simulink model "RL_Traction_motor"  (R2023a)
settings: Solver=VariableStepAuto  StartTime=0.0  StopTime=0.25  RelTol=1e-3
model workspace (MAT data in the model file):
  Cdc = 0.001
  Jm = 0.1234
  Ki_id = 710.3004
  Ki_iq = 1061.5
  Ki_omega = 500
  Kp_id = 0.8779
  Kp_iq = 1.0744
  Kp_omega = 20
  L0 = 0.00012184
  Ld = 0.00024368
  LdMatrix = [0.000182 0.00018 0.000178 0.000177 0.000176 0.00017475 0.0001735 0.00017247 0.00017132 0.00016571 0.00016537 0.00016571 ... (735 elements, 21x35)]
  Lq = 0.00029758
  LqMatrix = [0.000217 0.000217 0.000217 0.000217 0.000217 0.0002145 0.000212 0.0002115 0.00021022 0.0002079 0.00020461 0.0002079 ... (735 elements, 21x35)]
  PmMatrix = [0.0363 0.0363 0.0363 0.0363 0.0363 0.0363 0.0363 0.0363 0.0363 0.0363 0.0363 0.0363 ... (735 elements, 21x35)]
  Pmax = 35000
  Rs = 0.010087
  Tmax = 200
  Ts = 5e-06
  Tsc = 0.0001
  V1 = 290
  Vnom = 325
  fsw = 10000
  idVec = [-250 -225 -200 -175 -150 -125 -100 -75 -50 -25 0 25 ... (21 elements, 1x21)]
  iqVec = [-425 -400 -375 -350 -325 -300 -275 -250 -225 -200 -175 -150 ... (35 elements, 1x35)]
  p = 8
  psim = 0.044
undefined symbols (not defined in the file or in its folder): ee_sli_rtmsupport, gcbh, idMatrix, Imax, iqMatrix, rpmVec, TqVec, VdcVec
libraries: fl_lib x19, nesl_utility x13, eeGeneralControl x9, slpidlib x7, ee_lib x6, simulink x3, eeTransforms x2, batteryecm_lib x1, eeDqVoltageLimiter x1, eePwmGeneratorTwoLevel x1, eeResolverToDigitalConverter x1
(part 2 of 3)

== system RL_Traction_motor/Sensing Vdc ==
  PS-Simulink Converter4 : nesl_utility/PS-Simulink Converter  PhysicalDomain=network_engine_domain  SubClassName=ps_output  LeftPortType=input  RightPortType=output  PseudoPeriodic=off  Frequencies=[]  VectorFormat=1-D array  Unit=V  AffineConversion=off
  Voltage Sensor : fl_lib/Electrical/Electrical Sensors/Voltage Sensor
  + : PMIOPort  Side=Left
  - : PMIOPort  Port=2  Side=Right
  tag scope: Vdc=global
  wires:
  PS-Simulink Converter4/1 -> [Vdc]
  connections:
  Voltage Sensor/LConn1 -- +/RConn1
  Voltage Sensor/RConn2 -- -/RConn1
  PS-Simulink Converter4/LConn1 -- Voltage Sensor/RConn1

== system RL_Traction_motor/Sensing iabc ==
  Current Sensor : ee_lib/Sensors & Transducers/Current Sensor (Three-Phase)
      settings: LogSimulationData=on
  PS-Simulink Converter : nesl_utility/PS-Simulink Converter  PhysicalDomain=network_engine_domain  SubClassName=ps_output  LeftPortType=input  RightPortType=output  PseudoPeriodic=off  Frequencies=[]  VectorFormat=1-D array  Unit=A  AffineConversion=off
  Sensor time lag : Subsystem  mask{Ti=1e-5}
      mask prompts: Ti "Sensor time constant:"
  1 : PMIOPort  Side=Left
  2 : PMIOPort  Port=2  Side=Right
  tag scope: iabc=global
  wires:
  PS-Simulink Converter/1 -> Sensor time lag/1(In1)
  Sensor time lag/1(Out1) -> [iabc]
  connections:
  1/RConn1 -- Current Sensor/LConn1
  2/RConn1 -- Current Sensor/RConn2
  Current Sensor/RConn1 -- PS-Simulink Converter/LConn1

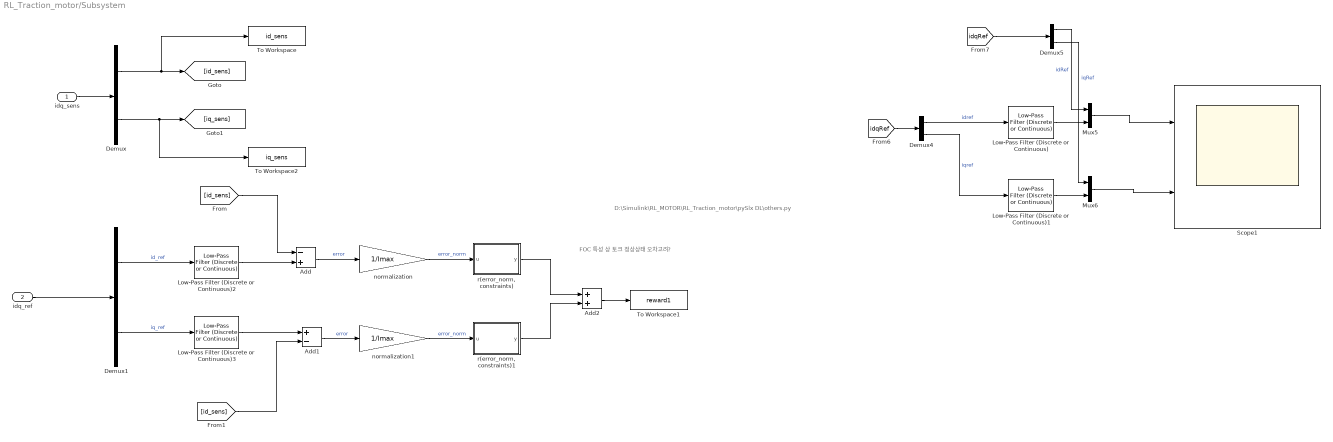
== system RL_Traction_motor/Subsystem ==
  note: D:\Simulink\RL_MOTOR\RL_Traction_motor\pySlx DL\others.py
  note: FOC 특성 상 토크 정상상태 오차고려?
  idq_sens : Inport
  idq_ref : Inport  Port=2
  Add : Sum  Inputs=-+
  Add1 : Sum  Inputs=+-
  Add2 : Sum
  Demux{,1,4..5} (4 alike) : Demux  Outputs=2
  Low-Pass Filter (Discrete or Continuous) : eeGeneralControl/Low-Pass Filter (Discrete or Continuous)  K=1  T=2.776235e-4  B=inf  A=-inf  init_option=Inherited from block input  x0=0  Ts=-1
  Low-Pass Filter (Discrete or Continuous)1 : eeGeneralControl/Low-Pass Filter (Discrete or Continuous)  K=1  T=1/2338913  B=inf  A=-inf  init_option=Inherited from block input  x0=0  Ts=-1
  Low-Pass Filter (Discrete or Continuous)2 : eeGeneralControl/Low-Pass Filter (Discrete or Continuous)  K=1  T=2.776235e-4  B=inf  A=-inf  init_option=Inherited from block input  x0=0  Ts=-1
  Low-Pass Filter (Discrete or Continuous)3 : eeGeneralControl/Low-Pass Filter (Discrete or Continuous)  K=1  T=1/2338913  B=inf  A=-inf  init_option=Inherited from block input  x0=0  Ts=-1
  Mux5 : Mux  Inputs=2
  Mux6 : Mux  Inputs=2
  Scope1 : Scope  NumInputPorts=2
  To Workspace : ToWorkspace  VariableName=id_sens  SaveFormat=Timeseries  SampleTime=-1
  To Workspace1 : ToWorkspace  VariableName=reward1  SaveFormat=Timeseries  SampleTime=-1
  To Workspace2 : ToWorkspace  VariableName=iq_sens  SaveFormat=Timeseries  SampleTime=-1
  normalization : Gain  Gain=1/Imax
  normalization1 : Gain  Gain=1/Imax
  "r(error_norm, constraints)" : MATLAB Function  TreatAsAtomicUnit=on
  "r(error_norm, constraints)1" : MATLAB Function  TreatAsAtomicUnit=on
  wires:
  Mux5/1 -> Scope1/1
  Demux5/1 -> Mux5/1  "idRef"
  Low-Pass Filter (Discrete or Continuous)1/1 -> Mux6/2
  Mux6/1 -> Scope1/2
  Demux4/1 -> Low-Pass Filter (Discrete or Continuous)/1  "idref"
  [idqRef] -> Demux4/1
  Low-Pass Filter (Discrete or Continuous)/1 -> Mux5/2
  [idqRef] -> Demux5/1
  Demux4/2 -> Low-Pass Filter (Discrete or Continuous)1/1  "iqref"
  Demux5/2 -> Mux6/1  "iqRef"
  idq_sens/1 -> Demux/1
  idq_ref/1 -> Demux1/1
  Demux1/1 -> Low-Pass Filter (Discrete or Continuous)2/1  "id_ref"
  Demux1/2 -> Low-Pass Filter (Discrete or Continuous)3/1  "iq_ref"
  Demux/1 -> To Workspace/1, [id_sens]
  Demux/2 -> To Workspace2/1, [iq_sens]
  Low-Pass Filter (Discrete or Continuous)2/1 -> Add/2
  Low-Pass Filter (Discrete or Continuous)3/1 -> Add1/1
  Add/1 -> normalization/1  "error"
  normalization/1 -> "r(error_norm, constraints)"/1(u)  "error_norm"
  "r(error_norm, constraints)1"/1(y) -> Add2/2
  normalization1/1 -> "r(error_norm, constraints)1"/1(u)  "error_norm"
  Add1/1 -> normalization1/1  "error"
  Add2/1 -> To Workspace1/1
  "r(error_norm, constraints)"/1(y) -> Add2/1
  [id_sens] -> Add/1
  [id_sens] -> Add1/2

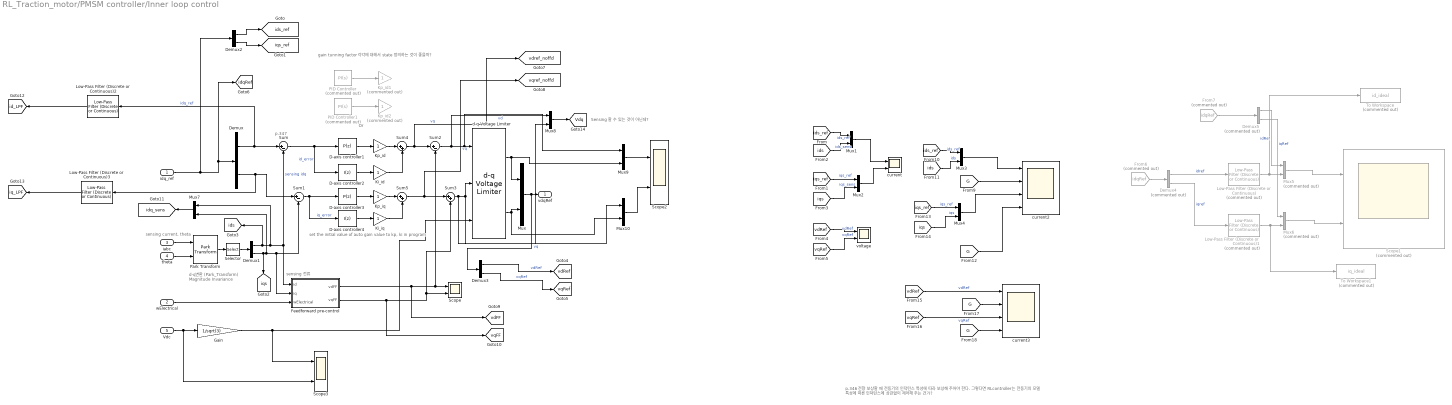
== system RL_Traction_motor/PMSM controller/Inner loop control ==
  note: Sensing 할 수 있는 것이 아닌데?
  note: gain tunning factor 각각에 대해서 state 정의하는 것이 좋을까?
  note: Or
  note: set the initial value of auto gain value to kp, ki in program
  note: p.346 전향 보상할 때 전동기의 인덕턴스 특성에 따라 보상해 주어야 한다.
      | 그렇다면 RLcontroller는 전동기의 모델 특성에 따른 인덕턴스에 상관없이 제어해 주는 건가?
  note: sensing current, theta
  note: p.347
  note: d-q변환
      | (Park_Transform)
      | Magnitude Invariance
  note: sensing 전류
  idq_ref : Inport
  wElectrical : Inport  Port=2
  iabc : Inport  Port=3
  theta : Inport  Port=4
  Vdc : Inport  Port=5
  D-axis controller1 : slpidlib/PID Controller  Controller=P  Form=Parallel  TimeDomain=Discrete-time  UseExternalTs=off  SampleTime=Tsc  IntegratorMethod=Forward Euler  FilterMethod=Forward Euler  ControllerParametersSource=internal  P=Kp_id  I="710.3          %710.3 (Ki_id)"  UseKiTs=off  D=0  N=100  UseFilter=on  TunerSelectOption=Transfer Function Based (PID Tuner App)  InitialConditionSource=internal  InitialConditionForIntegrator=0  InitialConditionForFilter=0  DifferentiatorICPrevScaledInput=0  ExternalReset=none  TrackingMode=off  Kt=1  LimitOutput=on  SatLimitsSource=internal  UpperSaturationLimit=Vnom/sqrt(3)  LowerSaturationLimit=-Vnom/sqrt(3)  LinearizeAsGain=on  AntiWindupMode=back-calculation  Kb=1000  LimitIntegrator=off  UpperIntegratorSaturationLimit=inf  LowerIntegratorSaturationLimit=-inf  POutMin=[]  POutMax=[]  IOutMin=[]  IOutMax=[]  DOutMin=[]  DOutMax=[]  NOutMin=[]  NOutMax=[]  SumOutMin=[]  SumOutMax=[]  SaturationOutMin=[]  SaturationOutMax=[]  PParamMin=[]  PParamMax=[]  IParamMin=[]  IParamMax=[]  DParamMin=[]  DParamMax=[]  NParamMin=[]  NParamMax=[]  KbParamMin=[]  KbParamMax=[]  KtParamMin=[]  KtParamMax=[]  KbOutMin=[]  KbOutMax=[]  KtOutMin=[]  KtOutMax=[]  IntegratorOutMin=[]  IntegratorOutMax=[]  FilterOutMin=[]  FilterOutMax=[]  SumI1OutMin=[]  SumI1OutMax=[]  SumI2OutMin=[]  SumI2OutMax=[]  SumI3OutMin=[]  SumI3OutMax=[]  SumI4OutMin=[]  SumI4OutMax=[]  SumDOutMin=[]  SumDOutMax=[]  DifferentiatorOutMin=[]  DifferentiatorOutMax=[]  FilterDiffOutCoefMin=[]  FilterDiffOutCoefMax=[]  ReciprocalOutMin=[]  ReciprocalOutMax=[]  SumDenOutMin=[]  SumDenOutMax=[]  SumNumOutMin=[]  SumNumOutMax=[]  DivideOutMin=[]  DivideOutMax=[]  UdiffTsProdOutMin=[]  UdiffTsProdOutMax=[]  NTsProdOutMin=[]  NTsProdOutMax=[]  UintegralTsProdOutMin=[]  UintegralTsProdOutMax=[]  UngainTsProdOutMin=[]  UngainTsProdOutMax=[]  ClampingZeroOutDataTypeStr=Inherit: Inherit via back propagation  ClampingZeroOutMin=[]  ClampingZeroOutMax=[]  FilterDenConstantOutDataTypeStr=Inherit: Inherit via back propagation  FilterDenConstantOutMin=[]  FilterDenConstantOutMax=[]  PCopyOutDataTypeStr=Inherit: Inherit via back propagation  PCopyOutMin=[]  PCopyOutMax=[]  NCopyOutDataTypeStr=Inherit: Inherit via back propagation  NCopyOutMin=[]  NCopyOutMax=[]  IntegratorContinuousStateAttributes=''  IntegratorStateMustResolveToSignalObject=off  IntegratorRTWStateStorageClass=Auto  FilterContinuousStateAttributes=''  FilterStateMustResolveToSignalObject=off  FilterRTWStateStorageClass=Auto  ParallelPVariant=InternalParameters  IdealPVariant=Disabled  IVariant=Disabled  DVariant=Disabled  IntegratorVariant=Disabled  SatVariant=Enabled  AWVariant=Disabled  PCopyVariant=Disabled  TRVariant=Disabled  FdbkBlocksVariant=Forward  IdealPFdbkVariant=Disabled  SatFdbkVariant=Disabled  DerivativeFilterVariant=Disabled  NVariant=Disabled  NCopyVariant=Disabled_SignalSpec  FilterICVariant=Disabled  IntegratorICVariant=Disabled  ExternalResetVariant=Disabled  TRSumVariant=Passthrough  SumFdbkVariant=Disabled  SumVariant=Passthrough_P  TsampFilterVariant=InternalTs  TsampNgainVariant=Passthrough  TsampIntegralVariant=Disabled_SignalSpec  ExternalSaturationOutDataTypeStr=Inherit: Same as second input
  D-axis controller2 : slpidlib/PID Controller  Controller=I  Form=Parallel  TimeDomain=Discrete-time  UseExternalTs=off  SampleTime=Tsc  IntegratorMethod=Forward Euler  FilterMethod=Forward Euler  ControllerParametersSource=internal  P="0.8779           %0.8779 (Kp_id)"  I=Ki_id  UseKiTs=off  D=0  N=100  UseFilter=on  TunerSelectOption=Transfer Function Based (PID Tuner App)  InitialConditionSource=internal  InitialConditionForIntegrator=0  InitialConditionForFilter=0  DifferentiatorICPrevScaledInput=0  ExternalReset=none  TrackingMode=off  Kt=1  LimitOutput=on  SatLimitsSource=internal  UpperSaturationLimit=Vnom/sqrt(3)  LowerSaturationLimit=-Vnom/sqrt(3)  LinearizeAsGain=on  AntiWindupMode=back-calculation  Kb=1000  LimitIntegrator=off  UpperIntegratorSaturationLimit=inf  LowerIntegratorSaturationLimit=-inf  POutMin=[]  POutMax=[]  IOutMin=[]  IOutMax=[]  DOutMin=[]  DOutMax=[]  NOutMin=[]  NOutMax=[]  SumOutMin=[]  SumOutMax=[]  SaturationOutMin=[]  SaturationOutMax=[]  PParamMin=[]  PParamMax=[]  IParamMin=[]  IParamMax=[]  DParamMin=[]  DParamMax=[]  NParamMin=[]  NParamMax=[]  KbParamMin=[]  KbParamMax=[]  KtParamMin=[]  KtParamMax=[]  KbOutMin=[]  KbOutMax=[]  KtOutMin=[]  KtOutMax=[]  IntegratorOutMin=[]  IntegratorOutMax=[]  FilterOutMin=[]  FilterOutMax=[]  SumI1OutMin=[]  SumI1OutMax=[]  SumI2OutMin=[]  SumI2OutMax=[]  SumI3OutMin=[]  SumI3OutMax=[]  SumI4OutMin=[]  SumI4OutMax=[]  SumDOutMin=[]  SumDOutMax=[]  DifferentiatorOutMin=[]  DifferentiatorOutMax=[]  FilterDiffOutCoefMin=[]  FilterDiffOutCoefMax=[]  ReciprocalOutMin=[]  ReciprocalOutMax=[]  SumDenOutMin=[]  SumDenOutMax=[]  SumNumOutMin=[]  SumNumOutMax=[]  DivideOutMin=[]  DivideOutMax=[]  UdiffTsProdOutMin=[]  UdiffTsProdOutMax=[]  NTsProdOutMin=[]  NTsProdOutMax=[]  UintegralTsProdOutMin=[]  UintegralTsProdOutMax=[]  UngainTsProdOutMin=[]  UngainTsProdOutMax=[]  ClampingZeroOutDataTypeStr=Inherit: Inherit via back propagation  ClampingZeroOutMin=[]  ClampingZeroOutMax=[]  FilterDenConstantOutDataTypeStr=Inherit: Inherit via back propagation  FilterDenConstantOutMin=[]  FilterDenConstantOutMax=[]  PCopyOutDataTypeStr=Inherit: Inherit via back propagation  PCopyOutMin=[]  PCopyOutMax=[]  NCopyOutDataTypeStr=Inherit: Inherit via back propagation  NCopyOutMin=[]  NCopyOutMax=[]  IntegratorContinuousStateAttributes=''  IntegratorStateMustResolveToSignalObject=off  IntegratorRTWStateStorageClass=Auto  FilterContinuousStateAttributes=''  FilterStateMustResolveToSignalObject=off  FilterRTWStateStorageClass=Auto  ParallelPVariant=Disabled  IdealPVariant=Disabled  IVariant=InternalParameters  DVariant=Disabled  IntegratorVariant=Discrete  SatVariant=Enabled  AWVariant=BackCalculation  PCopyVariant=Disabled  TRVariant=Disabled  FdbkBlocksVariant=Forward  IdealPFdbkVariant=Disabled  SatFdbkVariant=Disabled  DerivativeFilterVariant=Disabled  NVariant=Disabled  NCopyVariant=Disabled_SignalSpec  FilterICVariant=Disabled  IntegratorICVariant=InternalICs  ExternalResetVariant=Disabled  TRSumVariant=Passthrough  SumFdbkVariant=Disabled  SumVariant=Passthrough_I  TsampFilterVariant=InternalTs  TsampNgainVariant=Passthrough  TsampIntegralVariant=Disabled_SignalSpec  ExternalSaturationOutDataTypeStr=Inherit: Same as second input
  D-axis controller3 : slpidlib/PID Controller  Controller=P  Form=Parallel  TimeDomain=Discrete-time  UseExternalTs=off  SampleTime=Tsc  IntegratorMethod=Forward Euler  FilterMethod=Forward Euler  ControllerParametersSource=internal  P=Kp_iq  I="710.3          %710.3 (Ki_id)"  UseKiTs=off  D=0  N=100  UseFilter=on  TunerSelectOption=Transfer Function Based (PID Tuner App)  InitialConditionSource=internal  InitialConditionForIntegrator=0  InitialConditionForFilter=0  DifferentiatorICPrevScaledInput=0  ExternalReset=none  TrackingMode=off  Kt=1  LimitOutput=on  SatLimitsSource=internal  UpperSaturationLimit=Vnom/sqrt(3)  LowerSaturationLimit=-Vnom/sqrt(3)  LinearizeAsGain=on  AntiWindupMode=back-calculation  Kb=1000  LimitIntegrator=off  UpperIntegratorSaturationLimit=inf  LowerIntegratorSaturationLimit=-inf  POutMin=[]  POutMax=[]  IOutMin=[]  IOutMax=[]  DOutMin=[]  DOutMax=[]  NOutMin=[]  NOutMax=[]  SumOutMin=[]  SumOutMax=[]  SaturationOutMin=[]  SaturationOutMax=[]  PParamMin=[]  PParamMax=[]  IParamMin=[]  IParamMax=[]  DParamMin=[]  DParamMax=[]  NParamMin=[]  NParamMax=[]  KbParamMin=[]  KbParamMax=[]  KtParamMin=[]  KtParamMax=[]  KbOutMin=[]  KbOutMax=[]  KtOutMin=[]  KtOutMax=[]  IntegratorOutMin=[]  IntegratorOutMax=[]  FilterOutMin=[]  FilterOutMax=[]  SumI1OutMin=[]  SumI1OutMax=[]  SumI2OutMin=[]  SumI2OutMax=[]  SumI3OutMin=[]  SumI3OutMax=[]  SumI4OutMin=[]  SumI4OutMax=[]  SumDOutMin=[]  SumDOutMax=[]  DifferentiatorOutMin=[]  DifferentiatorOutMax=[]  FilterDiffOutCoefMin=[]  FilterDiffOutCoefMax=[]  ReciprocalOutMin=[]  ReciprocalOutMax=[]  SumDenOutMin=[]  SumDenOutMax=[]  SumNumOutMin=[]  SumNumOutMax=[]  DivideOutMin=[]  DivideOutMax=[]  UdiffTsProdOutMin=[]  UdiffTsProdOutMax=[]  NTsProdOutMin=[]  NTsProdOutMax=[]  UintegralTsProdOutMin=[]  UintegralTsProdOutMax=[]  UngainTsProdOutMin=[]  UngainTsProdOutMax=[]  ClampingZeroOutDataTypeStr=Inherit: Inherit via back propagation  ClampingZeroOutMin=[]  ClampingZeroOutMax=[]  FilterDenConstantOutDataTypeStr=Inherit: Inherit via back propagation  FilterDenConstantOutMin=[]  FilterDenConstantOutMax=[]  PCopyOutDataTypeStr=Inherit: Inherit via back propagation  PCopyOutMin=[]  PCopyOutMax=[]  NCopyOutDataTypeStr=Inherit: Inherit via back propagation  NCopyOutMin=[]  NCopyOutMax=[]  IntegratorContinuousStateAttributes=''  IntegratorStateMustResolveToSignalObject=off  IntegratorRTWStateStorageClass=Auto  FilterContinuousStateAttributes=''  FilterStateMustResolveToSignalObject=off  FilterRTWStateStorageClass=Auto  ParallelPVariant=InternalParameters  IdealPVariant=Disabled  IVariant=Disabled  DVariant=Disabled  IntegratorVariant=Disabled  SatVariant=Enabled  AWVariant=Disabled  PCopyVariant=Disabled  TRVariant=Disabled  FdbkBlocksVariant=Forward  IdealPFdbkVariant=Disabled  SatFdbkVariant=Disabled  DerivativeFilterVariant=Disabled  NVariant=Disabled  NCopyVariant=Disabled_SignalSpec  FilterICVariant=Disabled  IntegratorICVariant=Disabled  ExternalResetVariant=Disabled  TRSumVariant=Passthrough  SumFdbkVariant=Disabled  SumVariant=Passthrough_P  TsampFilterVariant=InternalTs  TsampNgainVariant=Passthrough  TsampIntegralVariant=Disabled_SignalSpec  ExternalSaturationOutDataTypeStr=Inherit: Same as second input
  D-axis controller4 : slpidlib/PID Controller  Controller=I  Form=Parallel  TimeDomain=Discrete-time  UseExternalTs=off  SampleTime=Tsc  IntegratorMethod=Forward Euler  FilterMethod=Forward Euler  ControllerParametersSource=internal  P="0.8779           %0.8779 (Kp_id)"  I=Ki_iq  UseKiTs=off  D=0  N=100  UseFilter=on  TunerSelectOption=Transfer Function Based (PID Tuner App)  InitialConditionSource=internal  InitialConditionForIntegrator=0  InitialConditionForFilter=0  DifferentiatorICPrevScaledInput=0  ExternalReset=none  TrackingMode=off  Kt=1  LimitOutput=on  SatLimitsSource=internal  UpperSaturationLimit=Vnom/sqrt(3)  LowerSaturationLimit=-Vnom/sqrt(3)  LinearizeAsGain=on  AntiWindupMode=back-calculation  Kb=1000  LimitIntegrator=off  UpperIntegratorSaturationLimit=inf  LowerIntegratorSaturationLimit=-inf  POutMin=[]  POutMax=[]  IOutMin=[]  IOutMax=[]  DOutMin=[]  DOutMax=[]  NOutMin=[]  NOutMax=[]  SumOutMin=[]  SumOutMax=[]  SaturationOutMin=[]  SaturationOutMax=[]  PParamMin=[]  PParamMax=[]  IParamMin=[]  IParamMax=[]  DParamMin=[]  DParamMax=[]  NParamMin=[]  NParamMax=[]  KbParamMin=[]  KbParamMax=[]  KtParamMin=[]  KtParamMax=[]  KbOutMin=[]  KbOutMax=[]  KtOutMin=[]  KtOutMax=[]  IntegratorOutMin=[]  IntegratorOutMax=[]  FilterOutMin=[]  FilterOutMax=[]  SumI1OutMin=[]  SumI1OutMax=[]  SumI2OutMin=[]  SumI2OutMax=[]  SumI3OutMin=[]  SumI3OutMax=[]  SumI4OutMin=[]  SumI4OutMax=[]  SumDOutMin=[]  SumDOutMax=[]  DifferentiatorOutMin=[]  DifferentiatorOutMax=[]  FilterDiffOutCoefMin=[]  FilterDiffOutCoefMax=[]  ReciprocalOutMin=[]  ReciprocalOutMax=[]  SumDenOutMin=[]  SumDenOutMax=[]  SumNumOutMin=[]  SumNumOutMax=[]  DivideOutMin=[]  DivideOutMax=[]  UdiffTsProdOutMin=[]  UdiffTsProdOutMax=[]  NTsProdOutMin=[]  NTsProdOutMax=[]  UintegralTsProdOutMin=[]  UintegralTsProdOutMax=[]  UngainTsProdOutMin=[]  UngainTsProdOutMax=[]  ClampingZeroOutDataTypeStr=Inherit: Inherit via back propagation  ClampingZeroOutMin=[]  ClampingZeroOutMax=[]  FilterDenConstantOutDataTypeStr=Inherit: Inherit via back propagation  FilterDenConstantOutMin=[]  FilterDenConstantOutMax=[]  PCopyOutDataTypeStr=Inherit: Inherit via back propagation  PCopyOutMin=[]  PCopyOutMax=[]  NCopyOutDataTypeStr=Inherit: Inherit via back propagation  NCopyOutMin=[]  NCopyOutMax=[]  IntegratorContinuousStateAttributes=''  IntegratorStateMustResolveToSignalObject=off  IntegratorRTWStateStorageClass=Auto  FilterContinuousStateAttributes=''  FilterStateMustResolveToSignalObject=off  FilterRTWStateStorageClass=Auto  ParallelPVariant=Disabled  IdealPVariant=Disabled  IVariant=InternalParameters  DVariant=Disabled  IntegratorVariant=Discrete  SatVariant=Enabled  AWVariant=BackCalculation  PCopyVariant=Disabled  TRVariant=Disabled  FdbkBlocksVariant=Forward  IdealPFdbkVariant=Disabled  SatFdbkVariant=Disabled  DerivativeFilterVariant=Disabled  NVariant=Disabled  NCopyVariant=Disabled_SignalSpec  FilterICVariant=Disabled  IntegratorICVariant=InternalICs  ExternalResetVariant=Disabled  TRSumVariant=Passthrough  SumFdbkVariant=Disabled  SumVariant=Passthrough_I  TsampFilterVariant=InternalTs  TsampNgainVariant=Passthrough  TsampIntegralVariant=Disabled_SignalSpec  ExternalSaturationOutDataTypeStr=Inherit: Same as second input
  Demux{,1..3} (4 alike) : Demux  Outputs=2
  Demux4 : Demux  Commented=on  Outputs=2
  Demux5 : Demux  Commented=on  Outputs=2
  Feedforward pre-control : Subsystem
  From6 : From  Commented=on  GotoTag=idqRef  TagVisibility=global
  From7 : From  Commented=on  GotoTag=idqRef  TagVisibility=global
  Gain : Gain  Gain=1/sqrt(3)
  Ki_id : Gain
  Ki_iq : Gain
  Kp_id : Gain
  Kp_id1 : Gain  Commented=on
  Kp_id2 : Gain  Commented=on
  Kp_iq : Gain
  Low-Pass Filter (Discrete or Continuous) : eeGeneralControl/Low-Pass Filter (Discrete or Continuous)  Commented=on  K=1  T=2.776235e-4  B=inf  A=-inf  init_option=Inherited from block input  x0=0  Ts=-1
  Low-Pass Filter (Discrete or Continuous)1 : eeGeneralControl/Low-Pass Filter (Discrete or Continuous)  Commented=on  K=1  T=1/2338913  B=inf  A=-inf  init_option=Inherited from block input  x0=0  Ts=-1
  Low-Pass Filter (Discrete or Continuous)2 : eeGeneralControl/Low-Pass Filter (Discrete or Continuous)  K=1  T=2.776235e-4  B=inf  A=-inf  init_option=Inherited from block input  x0=0  Ts=-1
  Low-Pass Filter (Discrete or Continuous)3 : eeGeneralControl/Low-Pass Filter (Discrete or Continuous)  K=1  T=1/2338913  B=inf  A=-inf  init_option=Inherited from block input  x0=0  Ts=-1
  Mux{,1..4,7..10} (9 alike) : Mux  Inputs=2
  Mux5 : Mux  Commented=on  Inputs=2
  Mux6 : Mux  Commented=on  Inputs=2
  PID Controller : slpidlib/PID Controller  Commented=on  Controller=PI  Form=Parallel  TimeDomain=Continuous-time  UseExternalTs=off  SampleTime=-1  IntegratorMethod=Forward Euler  FilterMethod=Forward Euler  ControllerParametersSource=internal  P=1  I=1  UseKiTs=off  D=0  N=100  UseFilter=on  TunerSelectOption=Transfer Function Based (PID Tuner App)  InitialConditionSource=internal  InitialConditionForIntegrator=0  InitialConditionForFilter=0  DifferentiatorICPrevScaledInput=0  ExternalReset=none  TrackingMode=off  Kt=1  LimitOutput=off  SatLimitsSource=internal  UpperSaturationLimit=inf  LowerSaturationLimit=-inf  LinearizeAsGain=on  AntiWindupMode=none  Kb=1  LimitIntegrator=off  UpperIntegratorSaturationLimit=inf  LowerIntegratorSaturationLimit=-inf  POutMin=[]  POutMax=[]  IOutMin=[]  IOutMax=[]  DOutMin=[]  DOutMax=[]  NOutMin=[]  NOutMax=[]  SumOutMin=[]  SumOutMax=[]  SaturationOutMin=[]  SaturationOutMax=[]  PParamMin=[]  PParamMax=[]  IParamMin=[]  IParamMax=[]  DParamMin=[]  DParamMax=[]  NParamMin=[]  NParamMax=[]  KbParamMin=[]  KbParamMax=[]  KtParamMin=[]  KtParamMax=[]  KbOutMin=[]  KbOutMax=[]  KtOutMin=[]  KtOutMax=[]  IntegratorOutMin=[]  IntegratorOutMax=[]  FilterOutMin=[]  FilterOutMax=[]  SumI1OutMin=[]  SumI1OutMax=[]  SumI2OutMin=[]  SumI2OutMax=[]  SumI3OutMin=[]  SumI3OutMax=[]  SumI4OutMin=[]  SumI4OutMax=[]  SumDOutMin=[]  SumDOutMax=[]  DifferentiatorOutMin=[]  DifferentiatorOutMax=[]  FilterDiffOutCoefMin=[]  FilterDiffOutCoefMax=[]  ReciprocalOutMin=[]  ReciprocalOutMax=[]  SumDenOutMin=[]  SumDenOutMax=[]  SumNumOutMin=[]  SumNumOutMax=[]  DivideOutMin=[]  DivideOutMax=[]  UdiffTsProdOutMin=[]  UdiffTsProdOutMax=[]  NTsProdOutMin=[]  NTsProdOutMax=[]  UintegralTsProdOutMin=[]  UintegralTsProdOutMax=[]  UngainTsProdOutMin=[]  UngainTsProdOutMax=[]  ClampingZeroOutDataTypeStr=Inherit: Inherit via back propagation  ClampingZeroOutMin=[]  ClampingZeroOutMax=[]  FilterDenConstantOutDataTypeStr=Inherit: Inherit via back propagation  FilterDenConstantOutMin=[]  FilterDenConstantOutMax=[]  PCopyOutDataTypeStr=Inherit: Inherit via back propagation  PCopyOutMin=[]  PCopyOutMax=[]  NCopyOutDataTypeStr=Inherit: Inherit via back propagation  NCopyOutMin=[]  NCopyOutMax=[]  IntegratorContinuousStateAttributes=''  IntegratorStateMustResolveToSignalObject=off  IntegratorRTWStateStorageClass=Auto  FilterContinuousStateAttributes=''  FilterStateMustResolveToSignalObject=off  FilterRTWStateStorageClass=Auto  ParallelPVariant=InternalParameters  IdealPVariant=Disabled  IVariant=InternalParameters  DVariant=Disabled  IntegratorVariant=Continuous  SatVariant=Disabled  AWVariant=Passthrough  PCopyVariant=Disabled  TRVariant=Disabled  FdbkBlocksVariant=Forward  IdealPFdbkVariant=Disabled  SatFdbkVariant=Disabled  DerivativeFilterVariant=Disabled  NVariant=Disabled  NCopyVariant=Disabled_SignalSpec  FilterICVariant=Disabled  IntegratorICVariant=InternalICs  ExternalResetVariant=Disabled  TRSumVariant=Passthrough  SumFdbkVariant=Disabled  SumVariant=Sum_PI  TsampFilterVariant=InternalTs  TsampNgainVariant=Passthrough  TsampIntegralVariant=Disabled_SignalSpec  ExternalSaturationOutDataTypeStr=Inherit: Same as second input
  PID Controller1 : slpidlib/PID Controller  Commented=on  Controller=PI  Form=Parallel  TimeDomain=Continuous-time  UseExternalTs=off  SampleTime=-1  IntegratorMethod=Forward Euler  FilterMethod=Forward Euler  ControllerParametersSource=internal  P=1  I=1  UseKiTs=off  D=0  N=100  UseFilter=on  TunerSelectOption=Transfer Function Based (PID Tuner App)  InitialConditionSource=internal  InitialConditionForIntegrator=0  InitialConditionForFilter=0  DifferentiatorICPrevScaledInput=0  ExternalReset=none  TrackingMode=off  Kt=1  LimitOutput=off  SatLimitsSource=internal  UpperSaturationLimit=inf  LowerSaturationLimit=-inf  LinearizeAsGain=on  AntiWindupMode=none  Kb=1  LimitIntegrator=off  UpperIntegratorSaturationLimit=inf  LowerIntegratorSaturationLimit=-inf  POutMin=[]  POutMax=[]  IOutMin=[]  IOutMax=[]  DOutMin=[]  DOutMax=[]  NOutMin=[]  NOutMax=[]  SumOutMin=[]  SumOutMax=[]  SaturationOutMin=[]  SaturationOutMax=[]  PParamMin=[]  PParamMax=[]  IParamMin=[]  IParamMax=[]  DParamMin=[]  DParamMax=[]  NParamMin=[]  NParamMax=[]  KbParamMin=[]  KbParamMax=[]  KtParamMin=[]  KtParamMax=[]  KbOutMin=[]  KbOutMax=[]  KtOutMin=[]  KtOutMax=[]  IntegratorOutMin=[]  IntegratorOutMax=[]  FilterOutMin=[]  FilterOutMax=[]  SumI1OutMin=[]  SumI1OutMax=[]  SumI2OutMin=[]  SumI2OutMax=[]  SumI3OutMin=[]  SumI3OutMax=[]  SumI4OutMin=[]  SumI4OutMax=[]  SumDOutMin=[]  SumDOutMax=[]  DifferentiatorOutMin=[]  DifferentiatorOutMax=[]  FilterDiffOutCoefMin=[]  FilterDiffOutCoefMax=[]  ReciprocalOutMin=[]  ReciprocalOutMax=[]  SumDenOutMin=[]  SumDenOutMax=[]  SumNumOutMin=[]  SumNumOutMax=[]  DivideOutMin=[]  DivideOutMax=[]  UdiffTsProdOutMin=[]  UdiffTsProdOutMax=[]  NTsProdOutMin=[]  NTsProdOutMax=[]  UintegralTsProdOutMin=[]  UintegralTsProdOutMax=[]  UngainTsProdOutMin=[]  UngainTsProdOutMax=[]  ClampingZeroOutDataTypeStr=Inherit: Inherit via back propagation  ClampingZeroOutMin=[]  ClampingZeroOutMax=[]  FilterDenConstantOutDataTypeStr=Inherit: Inherit via back propagation  FilterDenConstantOutMin=[]  FilterDenConstantOutMax=[]  PCopyOutDataTypeStr=Inherit: Inherit via back propagation  PCopyOutMin=[]  PCopyOutMax=[]  NCopyOutDataTypeStr=Inherit: Inherit via back propagation  NCopyOutMin=[]  NCopyOutMax=[]  IntegratorContinuousStateAttributes=''  IntegratorStateMustResolveToSignalObject=off  IntegratorRTWStateStorageClass=Auto  FilterContinuousStateAttributes=''  FilterStateMustResolveToSignalObject=off  FilterRTWStateStorageClass=Auto  ParallelPVariant=InternalParameters  IdealPVariant=Disabled  IVariant=InternalParameters  DVariant=Disabled  IntegratorVariant=Continuous  SatVariant=Disabled  AWVariant=Passthrough  PCopyVariant=Disabled  TRVariant=Disabled  FdbkBlocksVariant=Forward  IdealPFdbkVariant=Disabled  SatFdbkVariant=Disabled  DerivativeFilterVariant=Disabled  NVariant=Disabled  NCopyVariant=Disabled_SignalSpec  FilterICVariant=Disabled  IntegratorICVariant=InternalICs  ExternalResetVariant=Disabled  TRSumVariant=Passthrough  SumFdbkVariant=Disabled  SumVariant=Sum_PI  TsampFilterVariant=InternalTs  TsampNgainVariant=Passthrough  TsampIntegralVariant=Disabled_SignalSpec  ExternalSaturationOutDataTypeStr=Inherit: Same as second input
  Park Transform : eeTransforms/Park Transform  AxisAlignment=Q-axis  PowerInvariant=off
  Scope : Scope  NumInputPorts=2
  Scope1 : Scope  Commented=on  NumInputPorts=2
  Scope2 : Scope  NumInputPorts=2
  Scope3 : Scope  NumInputPorts=2
  Selector : Selector  InputPortWidth=3  IndexOptions=Index vector (dialog)  Indices=[1 2]  OutputSizes=1
  Sum : Sum  Inputs=|+-
  Sum1 : Sum  Inputs=|+-
  Sum2 : Sum  Inputs=|+-
  Sum3 : Sum  Inputs=|++
  Sum4 : Sum  Inputs=|++
  Sum5 : Sum  Inputs=|++
  To Workspace : ToWorkspace  Commented=on  VariableName=id_ideal  SampleTime=-1
      settings: Save2DSignal=2-D array (concatenate along first dimension)
  To Workspace1 : ToWorkspace  Commented=on  VariableName=iq_ideal  SampleTime=-1
      settings: Save2DSignal=2-D array (concatenate along first dimension)
  current : Scope  NumInputPorts=2
  current2 : Scope  NumInputPorts=4
  current3 : Scope  NumInputPorts=4
  d-q Voltage Limiter : eeDqVoltageLimiter/d-q Voltage Limiter  AxisPrio=Q-axis  Ts=Tsc
  voltage : Scope  NumInputPorts=2
  vdqRef : Outport  VectorParamsAs1DForOutWhenUnconnected=off
  tag scope: Vdq=global, id_LPF=global, idqRef=global, idq_sens=global, ids=global, ids_ref=global, iq_LPF=global, iqs=global, iqs_ref=global, vdFF=global, vdRef=global, vdref_noffd=global, vqFF=global, vqRef=global, vqref_noffd=global
  wires:
  Vdc/1 -> Scope3/2, Gain/1
  theta/1 -> Park Transform/2
  iabc/1 -> Park Transform/1
  Park Transform/1 -> Selector/1
  Gain/1 -> Scope3/1, d-q Voltage Limiter/3
  Feedforward pre-control/2(vqFF) -> [vqFF], Scope/2, Sum3/2
  Demux/1 -> Low-Pass Filter (Discrete or Continuous)2/1, Sum/1  "idq_ref"
  Demux1/1 -> [ids], Mux7/1, Feedforward pre-control/1(id), Sum/2  "sensing idq"
  Demux/2 -> Low-Pass Filter (Discrete or Continuous)3/1, Sum1/1
  idq_ref/1 -> Demux2/1, [idqRef], Demux/1
  wElectrical/1 -> Feedforward pre-control/3(wElectrical)
  d-q Voltage Limiter/2 -> Mux10/2, Mux/2
  d-q Voltage Limiter/1 -> Mux9/2, Mux/1
  Sum2/1 -> Mux8/1, Mux9/1, d-q Voltage Limiter/1  "vd"
  Selector/1 -> Demux1/1
  Mux/1 -> Demux3/1, vdqRef/1
  Sum3/1 -> Mux8/2, Mux10/1, d-q Voltage Limiter/2  "vq"
  Feedforward pre-control/1(vdFF) -> Sum2/2, Scope/1, [vdFF]
  Demux1/2 -> Feedforward pre-control/2(iq), Sum1/2, Mux7/2, [iqs]
  Sum/1 -> D-axis controller2/1, D-axis controller1/1  "id_error"
  Sum1/1 -> D-axis controller4/1, D-axis controller3/1  "iq_error"
  Demux2/2 -> [iqs_ref]
  Demux2/1 -> [ids_ref]
  [ids_ref] -> Mux1/1  "ids_ref"
  [ids] -> Mux1/2  "ids_sens"
  [iqs_ref] -> Mux2/1  "iqs_ref"
  [iqs] -> Mux2/2  "iqs_sens"
  Mux1/1 -> current/1
  Mux2/1 -> current/2
  Demux3/1 -> [vdRef]  "vdRef"
  Demux3/2 -> [vqRef]  "vqRef"
  [vqRef] -> voltage/2  "vqRef"
  [vdRef] -> voltage/1  "vdRef"
  [G] -> current3/2
  [G] -> current2/4
  [vdRef] -> current3/1  "vdRef"
  [G] -> current2/2
  [vqRef] -> current3/3  "vqRef"
  Mux4/1 -> current2/3
  [iqs_ref] -> Mux4/1  "iqs_ref"
  [iqs] -> Mux4/2  "iqs"
  [G] -> current3/4
  [ids] -> Mux3/2  "ids"
  [ids_ref] -> Mux3/1  "ids_ref"
  Mux3/1 -> current2/1
  From6/1 -> Demux4/1
  Demux4/1 -> Low-Pass Filter (Discrete or Continuous)/1  "idref"
  Demux4/2 -> Low-Pass Filter (Discrete or Continuous)1/1  "iqref"
  From7/1 -> Demux5/1
  Low-Pass Filter (Discrete or Continuous)/1 -> To Workspace/1, Mux5/2
  Demux5/1 -> Mux5/1  "idRef"
  Low-Pass Filter (Discrete or Continuous)1/1 -> To Workspace1/1, Mux6/2
  Demux5/2 -> Mux6/1  "iqRef"
  Mux5/1 -> Scope1/1
  Mux6/1 -> Scope1/2
  Sum4/1 -> [vdref_noffd], Sum2/1  "vq"
  Sum5/1 -> [vqref_noffd], Sum3/1  "vq"
  D-axis controller1/1 -> Kp_id/1
  Kp_id/1 -> Sum4/1
  D-axis controller2/1 -> Ki_id/1
  Ki_id/1 -> Sum4/2
  D-axis controller3/1 -> Kp_iq/1
  Kp_iq/1 -> Sum5/1
  D-axis controller4/1 -> Ki_iq/1
  Ki_iq/1 -> Sum5/2
  Mux7/1 -> [idq_sens]
  PID Controller/1 -> Kp_id1/1
  PID Controller1/1 -> Kp_id2/1
  Low-Pass Filter (Discrete or Continuous)2/1 -> [id_LPF]
  Low-Pass Filter (Discrete or Continuous)3/1 -> [iq_LPF]
  Mux8/1 -> [Vdq]
  Mux9/1 -> Scope2/1
  Mux10/1 -> Scope2/2

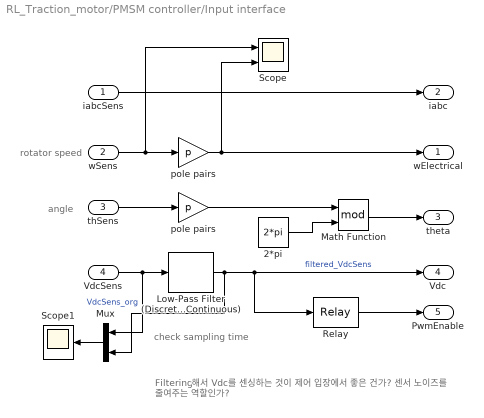
== system RL_Traction_motor/PMSM controller/Input interface ==
  note: angle
  note: rotator speed
  note: Filtering해서 Vdc를 센싱하는 것이 제어 입장에서 좋은 건가?
      | 센서 노이즈를 줄여주는 역할인가?
  note: check sampling time
  iabcSens : Inport
  wSens : Inport  Port=2
  thSens : Inport  Port=3
  VdcSens : Inport  Port=4
  2*pi : Constant  Value=2*pi  SampleTime=Tsc
  Low-Pass Filter (Discrete or Continuous) : eeGeneralControl/Low-Pass Filter (Discrete or Continuous)  K=1  T=0.001  B=inf  A=-inf  init_option=Inherited from block input  x0=0  Ts=Tsc
  Math Function : Math  Operator=mod  SignedPower=on
  Mux : Mux  Inputs=2
  Relay : Relay  OnSwitchValue=0.5*Vnom  OffSwitchValue=0.25*Vnom
  Scope : Scope  NumInputPorts=2
  Scope1 : Scope
  pole pairs : Gain  Gain=p
  "pole pairs " : Gain  Gain=p
  wElectrical : Outport  VectorParamsAs1DForOutWhenUnconnected=off
  iabc : Outport  Port=2  VectorParamsAs1DForOutWhenUnconnected=off
  theta : Outport  Port=3  VectorParamsAs1DForOutWhenUnconnected=off
  Vdc : Outport  Port=4  VectorParamsAs1DForOutWhenUnconnected=off
  PwmEnable : Outport  Port=5  VectorParamsAs1DForOutWhenUnconnected=off
  wires:
  VdcSens/1 -> Mux/1, Low-Pass Filter (Discrete or Continuous)/1  "VdcSens_org"
  Relay/1 -> PwmEnable/1
  Math Function/1 -> theta/1
  2*pi/1 -> Math Function/2
  "pole pairs "/1 -> Math Function/1
  iabcSens/1 -> iabc/1
  wSens/1 -> Scope/1, pole pairs/1
  thSens/1 -> "pole pairs "/1
  pole pairs/1 -> Scope/2, wElectrical/1
  Low-Pass Filter (Discrete or Continuous)/1 -> Mux/2, Vdc/1, Relay/1  "filtered_VdcSens"
  Mux/1 -> Scope1/1
